simulink model "flightControlSystem"  (R2023a)
settings: Solver=ode3  StartTime=0  StopTime=TFinal  FixedStep=Ts  RelTol=1e-3  EnableMultiTasking=on
undefined symbols (not defined in the file): afterTime, codertarget, COG_X, COG_Y, Controller, corner_step, degree_range1, degree_range2, degree_range3, DiscIntNeverNeededParam, Discrete, epsilon, Estimator, g, Gamma, gray, init, modi_PI, num_threshold, over_step, prev_degree_range, prev_degree_range2, Q, R, radius, radius2, ROI_Size, rotation_degree, rotation_degree2, Sensors, straight_step, strel, Time, Ts, tuning1, tuning11, tuning2, var_acc_angle_N, var_bias_gyr_N, var_gyro_p_N, Vehicle
libraries: simulink x41, slpidlib x4, ctrlSharedLib x4, visiontransforms x4, visiontextngfix x4, sharedtransform x3, visionanalysis x3, simulink_need_slupdate x1, parrotlib x1, visionmorphops x1
(part 3 of 4)

== system flightControlSystem/Control System/State Estimator/XY Position Estimator/EstimatorXYPosition ==
  note: Switching from orientationControl to Position
      | control reset the current world position estimate
      | (happens when using no markers)
  dxy_estimin : Inport
  orient_estimin : Inport  Port=2  SampleTime=Ts
  controlModePosVSOrient_flagin : Inport  Port=3
  dz_estimin : Inport  Port=4
  Math Function : Math  Operator=transpose  SignedPower=on
  Mux2 : Mux  Inputs=2
  Product : Product  Multiplication=Matrix(*)
  Rotation Angles to Direction Cosine Matrix : sharedtransform/Rotation Angles to Direction Cosine Matrix  rotationOrder=ZYX  aMode=aMode
  SelectdXY : Selector  InputPortWidth=3  IndexOptions=Index vector (dialog)  Indices=[1 2]  OutputSizes=1
  SimplyIntegrateVelocity : DiscreteIntegrator  ExternalReset=rising  SampleTime=Ts  ICPrevOutput=DiscIntNeverNeededParam  ICPrevScaledInput=DiscIntNeverNeededParam
  XY_estimout : Outport  VectorParamsAs1DForOutWhenUnconnected=off
  wires:
  controlModePosVSOrient_flagin/1 -> SimplyIntegrateVelocity/2
  Product/1 -> SelectdXY/1
  Mux2/1 -> Product/2
  dz_estimin/1 -> Mux2/2
  SimplyIntegrateVelocity/1 -> XY_estimout/1
  dxy_estimin/1 -> Mux2/1
  orient_estimin/1 -> Rotation Angles to Direction Cosine Matrix/1
  Rotation Angles to Direction Cosine Matrix/1 -> Math Function/1
  SelectdXY/1 -> SimplyIntegrateVelocity/1
  Math Function/1 -> Product/1

== system flightControlSystem/Image Processing System/Subsystem/viewer/centroids viewer ==
  p : Inport
  In2 : Inport  Port=2
  MATLAB Function1 : MATLAB Function  TreatAsAtomicUnit=on
  MATLAB Function2 : MATLAB Function  TreatAsAtomicUnit=on
  To Workspace1 : ToWorkspace  VariableName=centroids  SampleTime=-1
  To Workspace2 : ToWorkspace  VariableName=centroids_before  SampleTime=-1
  after : VideoViewer  colormapValue=gray(256)  FigPos=[3548 573 257 231]
  before : VideoViewer  colormapValue=gray(256)  FigPos=[3816 640 285 230]
  wires:
  In2/1 -> To Workspace1/1, MATLAB Function1/1(p)
  p/1 -> MATLAB Function2/1(p), To Workspace2/1
  MATLAB Function1/1(image) -> after/1
  MATLAB Function2/1(image) -> before/1

== system flightControlSystem/Image Processing System/corner detection subsystem1/straight line detector/center line viewer ==
  center_lines : Inport
  Constant : Constant  Value=zeros(120,160)
  Draw Shapes : visiontextngfix/Draw Shapes  shape=Lines  fill=off  lineWidth=1  fillClrSource=Specify via dialog  display=White  intensity=200  color=[100 100 100 100]  opacity=0.6  viewport=Entire image  antialiasing=off  inType=Obsolete  imagePorts=One multidimensional signal  roundingMode=Floor  overflowMode=off  memoryMode=Specify word length  memoryWordLength=16  prodOutputMode=Binary point scaling  prodOutputWordLength=32  prodOutputFracLength=14  memoryFracLength=15
  center lines : VideoViewer  colormapValue=gray(256)  FigPos=[987 659 418 304]
  wires:
  Draw Shapes/1 -> center lines/1
  Constant/1 -> Draw Shapes/1
  center_lines/1 -> Draw Shapes/2

== system flightControlSystem/Image Processing System/corner detection subsystem1/straight line detector/straight line viewer ==
  Pts : Inport
  Constant : Constant  Value=zeros(120,160)
  Draw Shapes : visiontextngfix/Draw Shapes  shape=Lines  fill=off  lineWidth=1  fillClrSource=Specify via dialog  display=White  intensity=200  color=[100 100 100 100]  opacity=0.6  viewport=Entire image  antialiasing=off  inType=Obsolete  imagePorts=One multidimensional signal  roundingMode=Floor  overflowMode=off  memoryMode=Specify word length  memoryWordLength=16  prodOutputMode=Binary point scaling  prodOutputWordLength=32  prodOutputFracLength=14  memoryFracLength=15
  Straight lines : VideoViewer  colormapValue=gray(256)  FigPos=[556 648 418 304]
  wires:
  Pts/1 -> Draw Shapes/2
  Constant/1 -> Draw Shapes/1
  Draw Shapes/1 -> Straight lines/1

== system flightControlSystem/Image Processing System/corner detection1/straight line detector/center line viewer ==
  center_lines : Inport
  Constant : Constant  Value=zeros(120,160)
  Draw Shapes : visiontextngfix/Draw Shapes  shape=Lines  fill=off  lineWidth=1  fillClrSource=Specify via dialog  display=White  intensity=200  color=[100 100 100 100]  opacity=0.6  viewport=Entire image  antialiasing=off  inType=Obsolete  imagePorts=One multidimensional signal  roundingMode=Floor  overflowMode=off  memoryMode=Specify word length  memoryWordLength=16  prodOutputMode=Binary point scaling  prodOutputWordLength=32  prodOutputFracLength=14  memoryFracLength=15
  center lines : VideoViewer  colormapValue=gray(256)  FigPos=[987 659 418 304]
  wires:
  center_lines/1 -> Draw Shapes/2
  Constant/1 -> Draw Shapes/1
  Draw Shapes/1 -> center lines/1

== system flightControlSystem/Image Processing System/corner detection1/straight line detector/straight line viewer ==
  Pts : Inport
  Constant : Constant  Value=zeros(120,160)
  Draw Shapes : visiontextngfix/Draw Shapes  shape=Lines  fill=off  lineWidth=1  fillClrSource=Specify via dialog  display=White  intensity=200  color=[100 100 100 100]  opacity=0.6  viewport=Entire image  antialiasing=off  inType=Obsolete  imagePorts=One multidimensional signal  roundingMode=Floor  overflowMode=off  memoryMode=Specify word length  memoryWordLength=16  prodOutputMode=Binary point scaling  prodOutputWordLength=32  prodOutputFracLength=14  memoryFracLength=15
  Straight lines : VideoViewer  colormapValue=gray(256)  FigPos=[556 648 418 304]
  wires:
  Draw Shapes/1 -> Straight lines/1
  Constant/1 -> Draw Shapes/1
  Pts/1 -> Draw Shapes/2

== system flightControlSystem/Control System/State Estimator/SensorPreprocessing/Temperature Compensation/Triggered Subsystem ==
  In1 : Inport
  Trigger : TriggerPort  TriggerType=either  VariantControl=Variant
  Out1 : Outport
  wires:
  In1/1 -> Out1/1

== system flightControlSystem/Control System/State Estimator/XY Position Estimator/EstimatorVelocity/AccelerationHandling ==
  dxy_estimin : Inport
  sensorIMU_datin : Inport  Port=2
  orient_estimin : Inport  Port=3
  Z_estimin : Inport  Port=4
  Add : Sum  Inputs=-+
  Bus Selector1 : BusSelector  OutputSignals=ddx,ddy,ddz
  Deactivate Acceleration If OF is not used due to low altitude : simulink/Logic and Bit Operations/Compare To Constant  relop=<=  const=Estimator.pos.opticalFlowZMax  OutDataTypeStr=boolean
  Logical Operator : Logic  Operator=OR  AllPortsSameDT=off  OutDataTypeStr=boolean
  Mux6 : Mux  Inputs=3
  Product : Product  Inputs=3
  Product1 : Product  Multiplication=Matrix(*)
  Rotation Angles to Direction Cosine Matrix : sharedtransform/Rotation Angles to Direction Cosine Matrix  rotationOrder=ZYX  aMode=aMode
  SelectPlanarddxy : Selector  InputPortWidth=3  IndexOptions=Index vector (dialog)  Indices=[1 2]  OutputSizes=1
  Selector : Selector  InputPortWidth=2  IndexOptions=Index vector (dialog)  Indices=1  OutputSizes=1
  Selector1 : Selector  InputPortWidth=2  IndexOptions=Index vector (dialog)  Indices=2  OutputSizes=1
  do not use acc if optical flow never available (Note OF@60Hz but ZOH to 200!) : simulink/Logic and Bit Operations/Compare To Constant  relop=~=  const=0  OutDataTypeStr=boolean
  do not use acc if optical flow never available (Note OF@60Hz but ZOH to 200!)1 : simulink/Logic and Bit Operations/Compare To Constant  relop=~=  const=0  OutDataTypeStr=boolean
  gainaccinput1 : Gain  OutDataTypeStr=single
  gravity : Constant  Value=[0 0 -g]
  acceleration_world : Outport  OutDataTypeStr=single  VectorParamsAs1DForOutWhenUnconnected=off
  wires:
  do not use acc if optical flow never available (Note OF@60Hz but ZOH to 200!)1/1 -> Logical Operator/2
  do not use acc if optical flow never available (Note OF@60Hz but ZOH to 200!)/1 -> Logical Operator/1
  Logical Operator/1 -> Product/1
  Selector1/1 -> do not use acc if optical flow never available (Note OF@60Hz but ZOH to 200!)1/1
  Selector/1 -> do not use acc if optical flow never available (Note OF@60Hz but ZOH to 200!)/1
  dxy_estimin/1 -> Selector1/1, Selector/1
  Product/1 -> acceleration_world/1
  Deactivate Acceleration If OF is not used due to low altitude/1 -> Product/3
  Z_estimin/1 -> Deactivate Acceleration If OF is not used due to low altitude/1
  Add/1 -> SelectPlanarddxy/1
  Product1/1 -> Add/1
  gravity/1 -> Product1/2
  SelectPlanarddxy/1 -> gainaccinput1/1
  Bus Selector1/3 -> Mux6/3  "<ddz>"
  Bus Selector1/1 -> Mux6/1  "<ddx>"
  sensorIMU_datin/1 -> Bus Selector1/1
  Mux6/1 -> Add/2
  Bus Selector1/2 -> Mux6/2  "<ddy>"
  orient_estimin/1 -> Rotation Angles to Direction Cosine Matrix/1
  Rotation Angles to Direction Cosine Matrix/1 -> Product1/1
  gainaccinput1/1 -> Product/2

== system flightControlSystem/Control System/State Estimator/XY Position Estimator/EstimatorVelocity/Angular velocity compensation for optical flow ==
  note: Optical flow readings are affected by both linear and angular velocity of the drone. We need to subtract the effect of angular velocity before using the flow data
  z_estimate : Inport
  Angular velocity w/o bias : Inport  Port=2
  Abs : Abs  SaturateOnIntegerOverflow=off
  Data Type Conversion : DataTypeConversion  SaturateOnIntegerOverflow=off  RndMeth=Floor
  Demux : Demux  Outputs=2
  Gain1 : Gain  Gain=-1
  Mux : Mux  Inputs=2
  Selector : Selector  InputPortWidth=3  IndexOptions=Index vector (dialog)  Indices=[1 2]  OutputSizes=1
  prod : Product  Inputs=**
  angular velocity correction : Outport
  wires:
  Gain1/1 -> Mux/1
  Mux/1 -> Data Type Conversion/1
  Demux/2 -> Gain1/1
  Data Type Conversion/1 -> angular velocity correction/1
  prod/1 -> Demux/1
  z_estimate/1 -> Abs/1
  Demux/1 -> Mux/2
  Selector/1 -> prod/2
  Abs/1 -> prod/1
  Angular velocity w/o bias/1 -> Selector/1

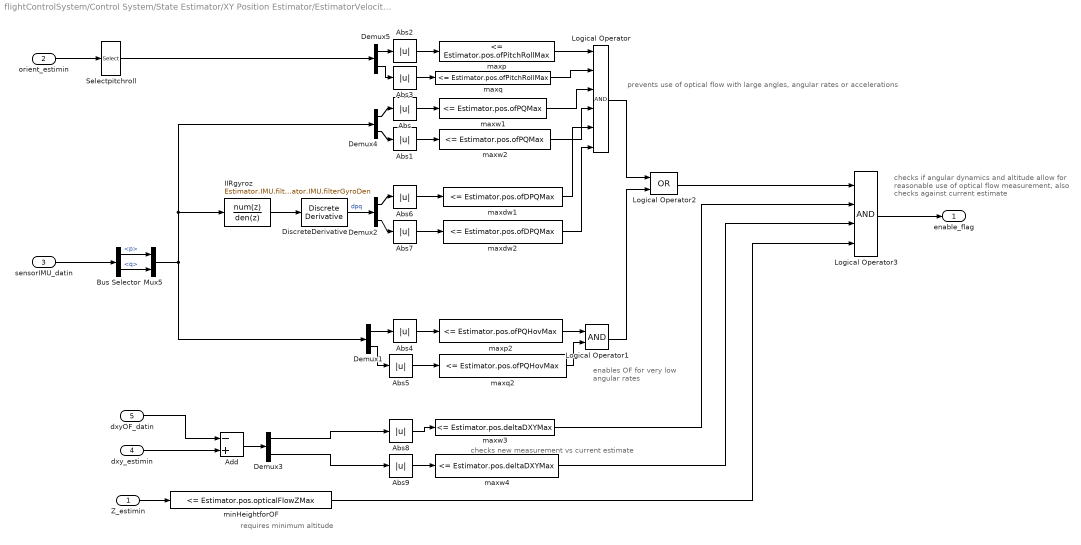
== system flightControlSystem/Control System/State Estimator/XY Position Estimator/EstimatorVelocity/DataHandling ==
  note: prevents use of optical flow with large angles, angular rates or accelerations
  note: enables OF for very
      | low angular rates
  note: checks if angular dynamics and altitude allow for
      | reasonable use of optical flow measurement,
      | also checks against current estimate
  note: checks new measurement vs current estimate
  note: requires minimum altitude
  Z_estimin : Inport
  orient_estimin : Inport  Port=2
  sensorIMU_datin : Inport  Port=3
  dxy_estimin : Inport  Port=4
  dxyOF_datin : Inport  Port=5
  Abs{,1..9} (10 alike) : Abs  SaturateOnIntegerOverflow=off
  Add : Sum  Inputs=-+
  Bus Selector : BusSelector  OutputSignals=p,q
  Demux{1..5} (5 alike) : Demux  Outputs=2
  DiscreteDerivative : simulink/Discrete/Discrete Derivative  gainval=1.0  ICPrevScaledInput=0.0  OutMin=[]  OutMax=[]  OutDataType=fixdt(1, 16)  OutScaling=2^-10  DoSatur=off
  IIRgyroz : DiscreteFilter  Numerator=Estimator.IMU.filterGyroNum  Denominator=Estimator.IMU.filterGyroDen
  Logical Operator : Logic  Inputs=6  AllPortsSameDT=off  OutDataTypeStr=boolean
  Logical Operator1 : Logic  AllPortsSameDT=off  OutDataTypeStr=boolean
  Logical Operator2 : Logic  Operator=OR  AllPortsSameDT=off  OutDataTypeStr=boolean
  Logical Operator3 : Logic  Inputs=4  AllPortsSameDT=off  OutDataTypeStr=boolean
  Mux5 : Mux  Inputs=2
  Selectpitchroll : Selector  InputPortWidth=3  IndexOptions=Index vector (dialog)  Indices=[2 3]  OutputSizes=1
  maxdw1 : simulink/Logic and Bit Operations/Compare To Constant  relop=<=  const=Estimator.pos.ofDPQMax  OutDataTypeStr=boolean
  maxdw2 : simulink/Logic and Bit Operations/Compare To Constant  relop=<=  const=Estimator.pos.ofDPQMax  OutDataTypeStr=boolean
  maxp : simulink/Logic and Bit Operations/Compare To Constant  relop=<=  const=Estimator.pos.ofPitchRollMax  OutDataTypeStr=boolean
  maxp2 : simulink/Logic and Bit Operations/Compare To Constant  relop=<=  const=Estimator.pos.ofPQHovMax  OutDataTypeStr=boolean
  maxq : simulink/Logic and Bit Operations/Compare To Constant  relop=<=  const=Estimator.pos.ofPitchRollMax  OutDataTypeStr=boolean
  maxq2 : simulink/Logic and Bit Operations/Compare To Constant  relop=<=  const=Estimator.pos.ofPQHovMax  OutDataTypeStr=boolean
  maxw1 : simulink/Logic and Bit Operations/Compare To Constant  relop=<=  const=Estimator.pos.ofPQMax  OutDataTypeStr=boolean
  maxw2 : simulink/Logic and Bit Operations/Compare To Constant  relop=<=  const=Estimator.pos.ofPQMax  OutDataTypeStr=boolean
  maxw3 : simulink/Logic and Bit Operations/Compare To Constant  relop=<=  const=Estimator.pos.deltaDXYMax  OutDataTypeStr=boolean
  maxw4 : simulink/Logic and Bit Operations/Compare To Constant  relop=<=  const=Estimator.pos.deltaDXYMax  OutDataTypeStr=boolean
  minHeightforOF : simulink/Logic and Bit Operations/Compare To Constant  relop=<=  const=Estimator.pos.opticalFlowZMax  OutDataTypeStr=boolean
  enable_flag : Outport  VectorParamsAs1DForOutWhenUnconnected=off
  wires:
  minHeightforOF/1 -> Logical Operator3/4
  IIRgyroz/1 -> DiscreteDerivative/1
  Mux5/1 -> Demux1/1, Demux4/1, IIRgyroz/1
  maxw4/1 -> Logical Operator3/3
  maxw3/1 -> Logical Operator3/2
  dxyOF_datin/1 -> Add/1
  Demux3/2 -> Abs9/1
  Demux3/1 -> Abs8/1
  dxy_estimin/1 -> Add/2
  Add/1 -> Demux3/1
  Abs9/1 -> maxw4/1
  Abs8/1 -> maxw3/1
  Logical Operator2/1 -> Logical Operator3/1
  Logical Operator3/1 -> enable_flag/1
  DiscreteDerivative/1 -> Demux2/1  "dpq"
  Demux2/2 -> Abs7/1
  Demux2/1 -> Abs6/1
  Abs7/1 -> maxdw2/1
  Abs6/1 -> maxdw1/1
  Logical Operator1/1 -> Logical Operator2/2
  Demux1/2 -> Abs5/1
  Demux1/1 -> Abs4/1
  Abs5/1 -> maxq2/1
  Abs4/1 -> maxp2/1
  Abs3/1 -> maxq/1
  Abs2/1 -> maxp/1
  Demux4/2 -> Abs1/1
  Demux4/1 -> Abs/1
  Abs1/1 -> maxw2/1
  Abs/1 -> maxw1/1
  Z_estimin/1 -> minHeightforOF/1
  Logical Operator/1 -> Logical Operator2/1
  maxw1/1 -> Logical Operator/3
  Bus Selector/1 -> Mux5/1  "<p>"
  Selectpitchroll/1 -> Demux5/1
  sensorIMU_datin/1 -> Bus Selector/1
  maxq2/1 -> Logical Operator1/2
  Bus Selector/2 -> Mux5/2  "<q>"
  maxp/1 -> Logical Operator/1
  maxw2/1 -> Logical Operator/4
  orient_estimin/1 -> Selectpitchroll/1
  maxdw1/1 -> Logical Operator/5
  maxdw2/1 -> Logical Operator/6
  maxq/1 -> Logical Operator/2
  Demux5/1 -> Abs2/1
  Demux5/2 -> Abs3/1
  maxp2/1 -> Logical Operator1/1

== system flightControlSystem/Control System/State Estimator/XY Position Estimator/EstimatorVelocity/xy velocity w//o angular velocity compensation ==
  note: Optical flow raw readings are converted to velocity in m/s based on the estimated altitude
  optical_flow : Inport
  z_estimate : Inport  Port=2
  " " : Product  Inputs=**
  Compare To Constant : simulink/Logic and Bit Operations/Compare To Constant  relop=<  const=200*4  OutDataTypeStr=boolean
  Counter Free-Running : simulink/Sources/Counter Free-Running  NumBits=32  tsamp=-1
  Gain : Gain  Gain=-1
  Select dxy : Selector  InputPortWidth=3  IndexOptions=Index vector (dialog)  Indices=[1 2]  OutputSizes=1
  Switch : Switch  Criteria=u2 > Threshold  SaturateOnIntegerOverflow=off  InputSameDT=off
  opticalFlowErrorCorrect : Gain  Gain=1.15
  optical_flow_dx_dy : Outport
  wires:
  Select dxy/1 -> optical_flow_dx_dy/1  "optical_flow_dx_dy"
  " "/1 -> opticalFlowErrorCorrect/1
  opticalFlowErrorCorrect/1 -> Switch/3
  Gain/1 -> " "/2
  Switch/1 -> Select dxy/1
  Counter Free-Running/1 -> Compare To Constant/1
  Compare To Constant/1 -> Switch/2
  optical_flow/1 -> " "/1, Switch/1
  z_estimate/1 -> Gain/1

== matlab function flightControlSystem/Image Processing System/Subsystem/calculate yaw ==
  data: u input; yaw output
function yaw = fcn(u)

p = u(2,:);

yaw = mod(atan2(p(2),p(1)) , 2*pi);

if yaw > pi
   yaw =  yaw- 2*pi; 
end

== matlab function flightControlSystem/Control System/Controller/Position Controller/Position error transformation (Earth to Body frame) ==
  data: yaw input; xy_err_earth input; xy_err_body output
function xy_err_body = fcn(yaw,xy_err_earth)

transformation = [cos(yaw), sin(yaw); -sin(yaw),  cos(yaw)];
xy_err_body = transformation * xy_err_earth;


end

== matlab function flightControlSystem/Image Processing System/Subsystem/viewer/centroids viewer/MATLAB Function1 ==
  data: p input; image output
function image = fcn(p)

image = zeros(120, 160);

for i = 1:5
    if( p(i,1) == 0)  || (p(i,2) == 0)
       continue; 
    end
    x = round(p(i,1));
    y = round(p(i,2));
    image(x,y) = 1;
end

== matlab function flightControlSystem/Image Processing System/Subsystem/viewer/centroids viewer/MATLAB Function2 ==
  data: p input; image output
function image = fcn(p)

image = zeros(120, 160);


for i = 1:5
    if( p(i,1) == 0)  || (p(i,2) == 0)
       continue; 
    end
    x = round(p(i,1));
    y = round(p(i,2));
    image(x,y) = 1;
end

== matlab function flightControlSystem/Control System/Path Planning/mpc/Triggered Subsystem/discrete_MPC ==
  data: input input; vx output; vy output; corner input; modi_PI input; R input; Q input; epsilon input; Gamma input; landing input; corner_step input; straight_step input
function [vx,vy]  = discrete_mpc(input,corner,modi_PI,R,Q,epsilon,Gamma, landing, corner_step, straight_step)
if landing==1
    vx=input(10);
    vy=input(11);
    return;
end


if corner==1
    step=corner_step;
else
    step=straight_step;
end
tic
%DISCRETE_MPC
% coder.extrinsic('quadprog');
%using drone dynamics
%result=[phi theta pi p q r u v w x y z];
Horizon =10;
x=input(1:12);
x_d=input(12+Horizon);
y_d=input(12+2*Horizon);
z_d=1.3;
dt=1;
desti=[0 0 0 0 0 0 0 0 0 x_d y_d z_d]';%destination
real_x=x(10);
real_y=x(11);
real_z=x(12);
dx=(x_d-real_x)/Horizon;
dy=(y_d-real_y)/Horizon;
dz=(z_d-real_z)/Horizon;
% reference making
desti_horizon=zeros(12*Horizon,1);
ref_const=zeros(12*Horizon,1);
for i=1:Horizon
    %    desti_horizon=[desti_horizon;[0 0 0 0 0 0 0 0 0 real_x+dx*i real_y+dy*i real_z+dz*i]'];
    desti_horizon(10+(i-1)*12)=x_d;
    desti_horizon(11+(i-1)*12)=y_d;
    desti_horizon(12+(i-1)*12)=z_d;
%     desti_horizon=[desti_horizon;[0 0 0 0 0 0 0 0 0 real_x+dx*(i) real_y+dy*(i) real_z+dz*(i)]'];
    ref_const(10+(i-1)*12)=input(12+i);
    ref_const(11+(i-1)*12)=input(12+Horizon+i);
end

%% quadprog

H=R+modi_PI'*Q*modi_PI;
f=((x)'*Gamma'*Q*modi_PI-desti_horizon'*Q*modi_PI);
xmax=repmat(1000000000,12*Horizon,1);
xmin=repmat(-100000000,12*Horizon,1);
u_max=repmat([10,10,10,10,10,10,10,10,10,1000,1000,1000,1,5,5,5]',Horizon,1);
u_min=repmat(-[10,10,10,50,50,50,50,50,50,1000,1000,1000,1,.001,.001,0.0011]',Horizon,1);
%U=quadprog(H,f',[eye(320);-eye(320);PI;-PI],[u_max;-u_min;(xmax)-Gamma*(x); (-xmin)+Gamma*(x)]);
temp_PI=zeros(Horizon*12,Horizon*16);
temp_ref=zeros(12*Horizon,1);
epsilon_r=zeros(12*Horizon,1);
for i=1:Horizon
    temp_PI(12*(i-1)+10,:)=modi_PI(12*(i-1)+10,:);
    temp_PI(12*(i-1)+11,:)=modi_PI(12*(i-1)+11,:);
    temp_PI(12*(i-1)+12,:)=modi_PI(12*(i-1)+12,:);
    temp_ref(12*(i-1)+10)=ref_const(12*(i-1)+10);
    temp_ref(12*(i-1)+11)=ref_const(12*(i-1)+11);
    temp_ref(12*(i-1)+12)=ref_const(12*(i-1)+12);
    epsilon_r(12*(i-1)+10)=epsilon(10);
    epsilon_r(12*(i-1)+11)=epsilon(11);
    epsilon_r(12*(i-1)+12)=epsilon(12);
end
temp_x=[0 0 0 0 0 0 0 0 0 x(10) x(11) 0]';
opts = optimoptions('quadprog','Algorithm','active-set');
% opts = optimoptions(opts,'MaxIterations',1e4); % Recommended
x0=zeros(16*Horizon,1);
% for i=1:Horizon
%    x0(1+16*(i-1))=x_esti(1);
%    x0(2+16*(i-1))=x_esti(2);
%    x0(3+16*(i-1))=x_esti(3);
%    x0(4+16*(i-1))=x_esti(4);
%    x0(5+16*(i-1))=x_esti(5);
%    x0(6+16*(i-1))=x_esti(6);
%    x0(7+16*(i-1))=x_esti(7);
%    x0(8+16*(i-1))=x_esti(8);
%    x0(9+16*(i-1))=x_esti(9);
%    x0(10+16*(i-1))=x_esti(10);
%    x0(11+16*(i-1))=x_esti(11);
%    x0(12+16*(i-1))=x_esti(12);
%    x0(13+16*(i-1))=0;
%    x0(14+16*(i-1))=0;
%    x0(15+16*(i-1))=0;
%    x0(16+16*(i-1))=0;
% end
for i=1:Horizon
   x0(1+16*(i-1))=x(1);
   x0(2+16*(i-1))=x(2);
   x0(3+16*(i-1))=x(3);
   x0(4+16*(i-1))=x(4);
   x0(5+16*(i-1))=x(5);
   x0(6+16*(i-1))=x(6);
   x0(7+16*(i-1))=x(7);
   x0(8+16*(i-1))=x(8);
   x0(9+16*(i-1))=x(9);
   x0(10+16*(i-1))=x(10);
   x0(11+16*(i-1))=x(11);
   x0(12+16*(i-1))=x(12);
   x0(13+16*(i-1))=0;
   x0(14+16*(i-1))=0;
   x0(15+16*(i-1))=0;
   x0(16+16*(i-1))=0;
end
U=zeros(16*Horizon,1);
U=quadprog(H,f',[eye(16*Horizon);-eye(16*Horizon);temp_PI;-temp_PI],[u_max;-u_min;(temp_ref+epsilon_r)-Gamma*(temp_x); (-(temp_ref-epsilon_r))+Gamma*(temp_x)],[],[],[],[],x0,opts);
y=zeros(12*Horizon,1);
y=Gamma*x+modi_PI*U;
a=12*step+10;
b=12*step+11;
vx = y(a);
vy = y(b);
toc
end

== stateflow chart flightControlSystem/Image Processing System/Chart ==
  state take_off
    entry:
    takeOffFlag= 0;
    refPosition1 = [0 0];
  state take_off_complete
    entry, during:
    [refPosition1, theta] = init(preprocessingDots);
    isStraightLine = 1;
  state straight_line_reference_generation
    entry:
    isLine = 1;
    during:
    tempPoint = zeros(1,2);
    [isLine, tempPoint, cutting_image] = sector_form(preprocessingDots, theta);
    [refPosition1, theta] = reference_generator(tempPoint);
    tempPoint2 =second_track_generator(preprocessingDots,  refPosition1);
    [refPosition2, theta2] = reference_generator(tempPoint2);
  state new_track_generation
    entry:
    isLine = 0;
    isLanding = 0;
    tempRef = zeros(1,2);
    during:
    state state_check
      [isLanding, tempRef,cntt,MAPP] = laning_check(ladingFlag, theta,landingDots);
    state asd
      tempPoint =track_generator(preprocessingDots,theta);
      [refPosition1, theta] = reference_generator(tempPoint);
      tempPoint2 =second_track_generator(preprocessingDots,  refPosition1);
      [refPosition2, theta2] = reference_generator(tempPoint2);
      isLine = 1;
    (default) -> state_check
    state_check -> asd
  state landing
    entry,during:
    during:
    %[isLanding, refPosition1,cntt,MAPP] = laning_check(ladingFlag, theta,landingDots);
    %refPosition2 = refPosition1;
    refPosition1=landingRef;
    refPosition2=landingRef;
  (default) -> take_off
  take_off -> take_off_complete : [abs(Z)  >  1.3]
  take_off_complete -> straight_line_reference_generation : [1]
  straight_line_reference_generation -> new_track_generation : after(afterTime,sec)[isLine == 0]
  new_track_generation -> straight_line_reference_generation [order 1] : [isLanding ==0 && isLine == 1]
  new_track_generation -> landing [order 2] : [isLanding == 1]
  data: points function_input; initial_ref function_output; initial_theta function_output; state function_output; ref function_output; points function_input; prev_theta function_input; MAP function_output; num_threshold parameter; degree_range1 parameter; points function_input; ref function_output; degree_range2 parameter; rotation_degree parameter; prev_degree_range parameter; radius parameter; prev_theta function_input; image function_input; dot function_input; point function_output; ref function_output; newTheta function_output; point function_input; points function_input; ref function_output; degree_range3 parameter; rotation_degree2 parameter; radius2 parameter; prev_degree_range2 parameter; rotationCenter function_input; flag function_input; curTheta function_input; state function_output; ref function_output; points function_input; COG_Y parameter; COG_X parameter; cnt function_output; MAP function_output; ROI_Size parameter; takeOffFlag local; refPosition1 output; refPosition2 output; preprocessingDots input; isLine local; COG_X constant double =60; COG_Y constant double =80; tempPoint local; ladingFlag input; theta local; tempPoint2 local; theta2 local; isLanding output; cutting_image output; Z input; tempRef local; isStraightLine local; afterTime parameter; landingDots input; cntt output; MAPP output; landingRef input
  function [initial_ref, initial_theta] = init(points):
    | function [initial_ref, initial_theta] = init(points)
    | 
    | % mean calculate
    | points(points==0) = NaN;
    | initial_ref = mean(points,1,'omitnan');
    | 
    | % cordinate change
    | initial_ref(1) = COG_X - initial_ref(1);
    | initial_ref(2) = initial_ref(2) - COG_Y;
    | 
    | % initial theta calculate
    | initial_theta = mod(atan2(initial_ref(2) ,initial_ref(1) ),2*pi);
  function [state,ref, MAP]= sector_form(points, prev_theta):
    | function [state,ref, MAP]= sector_form(points, prev_theta)
    | 
    | num_dots = size(points,1);
    | cutting_dots = zeros(num_dots,2);
    | ref = zeros(1,2);
    | cnt = 0;
    | MAP=zeros(120,160);
    | 
    | for i=1:num_dots
    |     %탈출조건
    |     if points(i,1) == 0
    |        break; 
    |     end
    |     % 0~180도 사이의 각만 추출
    |     delta = abs( mod(atan2(points(i,2)-COG_Y, COG_X-points(i,1)),2*pi)  -  prev_theta);
    |     if delta > pi
    |         delta = 2*pi - delta;
    |     end
    |     
    |     if  delta< deg2rad(degree_range1 * 0.5)
    |         cnt = cnt+1;
    |         cutting_dots(cnt,1) = points(i,1);
    |         cutting_dots(cnt,2) = points(i,2);
    |         MAP(points(i,1),points(i,2))=1;
    |     end
    | end
    | 
    | 
    | % %라벨 붙여서 해결하기
    | % pre_dist = Inf;
    | % center = ones(1,2);
    | % for i = 1:cnt
    | %     dist = norm( cutting_dots(i,:) - [COG_X, COG_Y]);
    | %     if dist < pre_dist
    | %         center = cutting_dots(i,:);
    | %         pre_dist = dist;
    | %     end
    | % end
    | % L_image = bwlabel(MAP,8);
    | % label = L_image(center(1,1), center(1,2) );
    | % seg_image = L_image==label;
    | % 
    | % cnt = 0;
    | % cutting_dots = zeros(num_dots,2);
    | % for i = 1:120
    | %    for j = 1:160
    | %       if  seg_image(i,j) == 1
    | %           cnt = cnt+1;
    | %           cutting_dots(cnt,1) = i;
    | %           cutting_dots(cnt,2) = j;
    | %       end
    | %    end
    | % end
    | cutting_dots(cutting_dots==0) = NaN;
    | ref = mean(cutting_dots,1,'omitnan');
    | 
    | % Line인지 아닌지 판단
    | if cnt > num_threshold
    |     state = 1;
    | else
    |     state = 0;
    | end
    | 
    | % if cnt > straight_threshold
    | %     straight_state = 1;
    | % else
    | %     straight_state = 0;
    | % end
    | 
    | 
    | 
    | % cutting_dots(cutting_dots==0) = NaN;
    | % rho = 4*2; % tunning
    | % diagonal = 100;
    | % iterator = ceil(diagonal/rho);
    | % R = 5; %tunning
    | % theta = pi - prev_theta; % frame좌표로 변환
    | % P = zeros(1,2);
    | % cornerFalg = 0;
    | % radius = 0;
    | % for k = 0:iterator
    | %      P = [COG_X, COG_Y] + k * [rho*cos(prev_theta), rho*sin(prev_theta)];
    | %      if isempty( rangesearch(cutting_dots,P,R) )
    | %          radius = rho*k;
    | %      end
    | % end
    | % 
    | % num = 0;
    | % for i=1:cnt
    | %     % NaN때문에 여기서 에러 날수도?
    | %     if isnan(cutting_dots(i,:))
    | %        break; 
    | %     end
    | %    if norm(cutting_dots(i,:) - [COG_X, COG_Y]) > radius
    | %        cutting_dots(i,:) = NaN;
    | %        num = num + 1;
    | %    end
    | % end
    | % ref = mean(cutting_dots,1,'omitnan');
    | % 
    | % cnt = cnt - num;
    | % if cnt > num_threshold
    | %     state = 1;
    | % else
    | %     state = 0;
    | % end
    | % %여기서 state = 0이 계속 타지네... 흠흠..!@#!@#@!#!
    | 
    | 
    | 
    | 
    | % % % se = strel('disk',3);
    | % % % MAP = imdilate(MAP, se);
    | % % % pre_dist = Inf;
    | % % % center = ones(1,2);
    | % % % for i = 1:cnt
    | % % %     dist = norm( cutting_dots(i,:) - [COG_X, COG_Y]);
    | % % %     if dist < pre_dist
    | % % %         center = cutting_dots(i,:);
    | % % %         pre_dist = dist;
    | % % %     end
    | % % % end
    | % % % L_image = bwlabel(MAP,8);
    | % % % label = L_image(center(1,1), center(1,2) );
    | % % % seg_image = L_image==label;
    | % % % 
    | % % % cnt = 0;
    | % % % cutting_dots = zeros(num_dots,2);
    | % % % for i = 1:120
    | % % %    for j = 1:160
    | % % %       if  seg_image(i,j) == 1
    | % % %           cnt = cnt+1;
    | % % %           cutting_dots(cnt,1) = i;
    | % % %           cutting_dots(cnt,2) = j;
    | % % %       end
    | % % %    end
    | % % % end
    | % % % cutting_dots(cutting_dots==0) = NaN;
    | % % % ref = mean(cutting_dots,1,'omitnan');
    | % % 
    | % % 
    | % % % I = find(seg_image==1);
    | % % % [row, col] = ind2sub(size(seg_image), I);
    | % % % dotss = zeros(2000,2);
    | % % % for i= 1:size(row)
    | % % %     dotss = [row(i), col(i)];
    | % % % end
    | % % % dotss(dotss==0) = NaN;
    | % % % ref = mean(dotss,1,'omitnan');
    | % % 
    | % % 
    | % % % 일정한 호 이내의 점 추출 (방법이 잘못 된듯)
    | % % % r1 = 20;
    | % % % r2 = 30;
    | % % % arcPoints = zeros(100,2);
    | % % % idx = 1;
    | % % % for i = 1:num_dots
    | % % %     if cutting_dots(i,1) == 0
    | % % %        break; 
    | % % %     end
    | % % %     R = sqrt( (cutting_dots(i,1) - COG_X)^2 + (cutting_dots(i,2) - COG_Y)^2 ) ;
    | % % %     if R>=r1 && R<=r2
    | % % %         arc_cnt = arc_cnt + 1;
    | % % %     end
    | % % %     if R <= r1
    | % % %         arcPoints(idx,1) = cutting_dots(i,1);
    | % % %         arcPoints(idx,2) = cutting_dots(i,2);
    | % % %         idx = idx+1;
    | % % %     end  
    | % % % end
    | % % % 
    | % % % if arc_cnt > arc_threshold
    | % % %     cutting_dots(cutting_dots==0) = NaN;
    | % % %     ref = mean(cutting_dots,1,'omitnan');
    | % % % else
    | % % %     arcPoints(arcPoints==0) = NaN;
    | % % %     ref = mean(arcPoints,1,'omitnan');
    | % % % end
    | % % 
    | % % 
    | % % % % clustering
    | % % % temp_dist = 0;
    | % % % p = zeros(1,2);
    | % % % center = [60, 80];
    | % % % for i = 1:num_dots
    | % % %     if cutting_dots(i,1) == 0
    | % % %         break;
    | % % %     end
    | % % %    dist = norm( center - cutting_dots(1,:) );  
    | % % %    if dist > temp_dist
    | % % %        p = cutting_dots(i,:);
    | % % %        temp_dist = dist;
    | % % %    end
    | % % % end
    | % % % centroids = [center ; p];
    | % % % idx = knnsearch(centroids,cutting_dots);
    | % % % cutting_dots(cutting_dots==0) = NaN;
    | % % % ref = mean(cutting_dots(idx==1,:),1,'omitnan');
  function ref  = track_generator(points, prev_theta):
    | function ref  = track_generator(points, prev_theta)
    | num_dots = size(points,1);
    | cutting_dots = zeros(num_dots,2);
    | iterator = round(360 / rotation_degree);
    | prev_theta = mod(prev_theta+ pi , 2*pi);
    | 
    | cnt = 1;
    | ref = zeros(1,2);
    | plus_degree = (prev_degree_range/2) + (degree_range2/2);
    | iterator = round( (360 - 2*plus_degree) / rotation_degree );
    | pre_cnt = 0;
    | for i = 0:iterator
    |     cutting_dots = zeros(num_dots,2);
    |     cnt = 0;
    |     for j=1:num_dots
    |         %탈출조건
    |         if points(j,1) == 0
    |            break;
    |         end
    |         % 0~180도 사이의 각만 추출
    |         %delta = abs( mod(atan2(points(j,2)-COG_Y, COG_X-points(j,1)),2*pi)  -  mod(prev_theta + i*deg2rad(rotation_degree) , 2*pi) );
    |         delta = abs( mod(atan2(points(j,2)-COG_Y, COG_X-points(j,1)),2*pi)  -  mod(prev_theta + deg2rad(plus_degree) +i*deg2rad(rotation_degree) , 2*pi) );
    |         if delta > pi
    |             delta = 2*pi - delta;
    |         end
    |         R = sqrt( (points(j,1) - COG_X)^2 + (points(j,2) - COG_Y)^2 ) ;
    |         % degree_range 이내 && radius이내 점 추출
    |         if  delta< deg2rad(degree_range2 * 0.5) && R < radius
    |             cnt = cnt+1;
    |             cutting_dots(cnt,1) = points(j,1);
    |             cutting_dots(cnt,2) = points(j,2);
    |         end
    |     end
    |     if cnt > pre_cnt
    |         cutting_dots(cutting_dots==0) = NaN;
    |         ref = mean(cutting_dots,1,'omitnan');
    |         pre_cnt = cnt;
    |     end
    | end
  function point = means_circle(image, dot):
    | function point = means_circle(image, dot)
    | 
    | r = 30;
    | 
    | % dot을 pixel좌표로 변환
    | % dot(1) = COG_X - dot(1);
    | % dot(2) = dot(2) + COG_Y;
    | 
    | % boundary processing
    | if dot(1) -r < 1
    |    startX = 1;
    | else
    |     startX = dot(1) -r;
    | end
    |     
    | if dot(2) -r < 1
    |    startY = 1;
    | else
    |     startY = dot(2) -r;
    | end
    | 
    | if dot(1) + r > 120
    |     endX = 120;
    | else
    |     endX = dot(1) + r;
    | end
    | 
    | if dot(2) + r > 160
    |     endY = 160;
    | else
    |     endY = dot(2) + r;
    | end
    |     
    | startPonit = [startX, startY];
    | endPoint = [endX, endY];
    | 
    | % k-means
    | ROIdots = zeros(2000,2);
    | idx = 1;
    | 
    | for i = round(startX) : round(endX)
    |     for j = round(startY) : round(endY)
    |        if image(i,j) == 1
    |            dist = sqrt( (dot(1) - i)^2 + (dot(2) - j)^2  );
    |            if dist <= r
    |               ROIdots(idx,1) = i;
    |               ROIdots(idx,2) = j;
    |               idx = idx+1;
    |            end
    |        end
    |     end
    | end
    | 
    | ROIdots(ROIdots==0) = NaN;
    | point = mean(ROIdots,1,'omitnan');
  function [ref, newTheta] = reference_generator(point):
    | function [ref, newTheta] = reference_generator(point)
    | 
    | ref = zeros(1,2);
    | ref(1) = COG_X - point(1);
    | ref(2) = point(2) - COG_Y;
    | newTheta = mod(atan2(ref(2) ,ref(1) ),2*pi);
  function ref  = second_track_generator(points, rotationCenter):
    | function ref  = second_track_generator(points, rotationCenter)
    | 
    | num_dots = size(points,1);
    | cutting_dots = zeros(num_dots,2);
    | iterator = round(360 / rotation_degree2);
    | prev_theta = mod(atan2( 0 - rotationCenter(2) , 0 - rotationCenter(1) ),2*pi);
    | cnt = 1;
    | ref = zeros(1,2);
    | 
    | plus_degree = (prev_degree_range2/2) + (degree_range3/2); 
    | iterator = round( (360 - 2*plus_degree) / rotation_degree2 );
    | 
    | 
    | pre_cnt = 0;
    | for i = 0:iterator
    |     cutting_dots = zeros(num_dots,2);
    |     cnt = 1;
    |     for j=1:num_dots
    |         %탈출조건
    |         if points(j,1) == 0
    |            break; 
    |         end
    |         % 0~180도 사이의 각만 추출
    |         P = [COG_X-points(j,1), points(j,2)-COG_Y];
    |         delta = abs( mod(atan2(P(2) - rotationCenter(2) , P(1) - rotationCenter(1) ),2*pi)  -  mod(prev_theta + deg2rad(plus_degree) +i*deg2rad(rotation_degree2) , 2*pi) );
    |         if delta > pi
    |             delta = 2*pi - delta;
    |         end
    |         R = sqrt( (P(1) - rotationCenter(1))^2 + (P(2) - rotationCenter(2))^2 ) ;
    |         % degree_range 이내 && radius이내 점 추출
    |         if  delta< deg2rad(degree_range3 * 0.5) && R < radius2
    |             cutting_dots(cnt,1) = points(j,1);
    |             cutting_dots(cnt,2) = points(j,2);
    |             cnt = cnt+1;
    |         end
    |     end
    |     
    |     if cnt > pre_cnt 
    |         cutting_dots(cutting_dots==0) = NaN;
    |         ref = mean(cutting_dots,1,'omitnan');
    |         pre_cnt = cnt;
    |     end
    |     
    | end
  function [state, ref,cnt, MAP] = laning_check(flag, curTheta, points):
    | function [state, ref,cnt, MAP] = laning_check(flag, curTheta, points)
    | 
    | num_dots = size(points,1);
    | cutting_dots = zeros(num_dots,2);
    | ref = zeros(1,2);
    | cnt = 0;
    | landing_threshold = 10;
    | MAP=zeros(120,160);
    | 
    | for i=1:num_dots
    |     %탈출조건
    |     if points(i,1) == 0
    |        break; 
    |     end
    |     % 0~180도 사이의 각만 추출
    |     delta = abs( mod(atan2(points(i,2)-(ROI_Size/2), (ROI_Size/2)-points(i,1)),2*pi)  -  curTheta);
    |     if delta > pi
    |         delta = 2*pi - delta;
    |     end
    |     
    |     if  delta< deg2rad(90 * 0.5)
    |         cnt = cnt+1;
    |         cutting_dots(cnt,1) = points(i,1);
    |         cutting_dots(cnt,2) = points(i,2);
    |         MAP(points(i,1),points(i,2))=1;
    |     end
    | end
    | 
    | 
    | state = 0;
    | 
    | if flag == 1 && cnt > landing_threshold
    |     cutting_dots(cutting_dots==0) = NaN;
    |     ref = mean(cutting_dots,1,'omitnan');
    |     ref(1) = (ROI_Size/2) - ref(1);
    |     ref(2) = ref(2) - (ROI_Size/2);
    |     
    |     state = 1;
    | else
    |     state = 0;
    | end
    | 
    | % landingTheta = mod(atan2(landing_ref(2), landing_ref(1)), 2*pi);
    | % deltaTheta = abs(mod(landingTheta - curTheta, 2*pi));
    | % if deltaTheta > pi
    | %             deltaTheta = 2*pi - deltaTheta;
    | % end
    | % 
    | % if flag == 1 && deltaTheta < deg2rad(30 * 0.5)
    | %     state = 1;
    | %     ref = landing_ref;
    | % end

== matlab function flightControlSystem/Image Processing System/preprocessing subsystem/Line segment ==
  data: dots input; MAP input; seg_image output; COG_X parameter; COG_Y parameter
function seg_image  = fcn(dots, MAP,COG_X, COG_Y)


num_dots = size(dots,1);

tmep_dist = Inf;
center = ones(1,2);
for i = 1:num_dots
    if dots(i,1) == 0
        break;
    end
    dist = norm( dots(i,:) - [COG_X, COG_Y]);
    if dist < tmep_dist
        center = dots(i,:);
        tmep_dist = dist;
    end
end


L_image = bwlabel(MAP,8);
label = L_image(center(1,1), center(1,2) );
seg_image = L_image==label;

cnt = 0;
cutting_dots = zeros(num_dots,2);
for i = 1:120
   for j = 1:160
      if  seg_image(i,j) == 1
          cnt = cnt+1;
          cutting_dots(cnt,1) = i;
          cutting_dots(cnt,2) = j;
      end
   end
end

== matlab function flightControlSystem/Image Processing System/Subsystem1/MATLAB Function2 ==
  data: X input; prev_points output; Y input; COG_X parameter; COG_Y parameter; MAP output
function [prev_points,MAP] = fcn(X, Y,COG_X, COG_Y)
persistent X1 X2 X3 Y1 Y2 Y3
if isempty(X1)
    X1 = 0;
end
if isempty(X2)
    X2 = 0;
end
if isempty(X3)
    X3 = 0;
end
if isempty(Y1)
    Y1 = 0;
end
if isempty(Y2)
    Y2 = 0;
end
if isempty(Y3)
    Y3 = 0;
end
prev_points = [COG_X-(X1-X)*2000 COG_Y+(Y1-Y)*2000;COG_X-(X2-X)*2000 COG_Y+(Y2-Y)*2000;COG_X-(X3-X)*2000 COG_Y+(Y3-Y)*2000];
prev_points = round(prev_points);
X3 = X2; Y3 = Y2;
X2 = X1; Y2 = Y1;
X1 = X; Y1 = Y;
MAP = zeros(120,160);
for i=1:3
    if 1<=prev_points(i,1) && prev_points(i,1)<=120 && 1<=prev_points(i,2) && prev_points(i,2)<=160 
        MAP(prev_points(i,1),prev_points(i,2))=1;
    end
end

== matlab function flightControlSystem/Image Processing System/preprocessing subsystem/preprocessing ==
  data: bin_image input; ref_image output; preporcessingDots output
function [ref_image, preporcessingDots]  = square_mean(bin_image)
%필요한 점들 뽑아내기 위한 변수들

rSize = 4;
threshold = 10;    
n = (120/rSize) * (160/rSize); 
ref_image = zeros(120,160);
preporcessingDots = zeros(n,2);
num_dots = 0;

for i=0:((120-rSize)/rSize)
    for j=0:((160-rSize)/rSize)
        if sum(bin_image(rSize*i+1:rSize*i+rSize, rSize*j+1:rSize*j+rSize),'all') > threshold
            ref_image(rSize*i+(rSize/2),rSize*j+(rSize/2))=1;
            num_dots = num_dots+1;
            preporcessingDots(num_dots,1) = rSize*i+(rSize/2);
            preporcessingDots(num_dots,2) = rSize*j+(rSize/2);
        end
    end
end

== matlab function flightControlSystem/Image Processing System/Result of previous work for backup/clustering ==
  data: centroids_before output; X input; centroids output
function [centroids_before,centroids] = fcn(X)



K = 5;
n = size(X, 1);
centroids = zeros(K,2);

% 1st 좌표
centroids(1,:) = [60, 80];

% 2nd  좌표 ,중앙에서 가장 먼 픽셀 찾기
d = 0;
for i = 1:n
   %temp_d = (60-X(i,1))^2  + (80-X(i,2))^2;
   temp_d = norm(centroids(1,:) - X(i,:) );
   if(temp_d > d && X(i,1) ~= 0)
      d= temp_d;
      centroids(2,1) = X(i,1);
      centroids(2,2) = X(i,2);
   end
end

% 3th 좌표
LS=100000;
for i = 1:n
    temp_d1 = norm(centroids(1,:)-X(i,:) );
    temp_d2 = norm(centroids(2,:)-X(i,:) );
    temp_LS = temp_d1^2 + temp_d2^2;
    if((temp_LS < LS) && X(i,1) ~= 0)
        LS = temp_LS;
        centroids(3,1) = X(i,1);
        centroids(3,2) = X(i,2);
   end
end

% 4th, 5th 좌표
LS=100000;
for i = 1:n
    temp_d1 = norm(centroids(1,:)-X(i,:) );
    temp_d3 = norm(centroids(3,:)-X(i,:) );
    temp_LS = temp_d1^2 +  temp_d3^2;
    if((temp_LS < LS) && X(i,1) ~= 0)
        LS = temp_LS;
        centroids(4,1) = X(i,1);
        centroids(4,2) = X(i,2);
    end
end
LS=100000;
for i = 1:n
    temp_d2 = norm(centroids(2,:)-X(i,:) );
    temp_d3 = norm(centroids(3,:)-X(i,:) );
    temp_LS = temp_d2^2 +  temp_d3^2;
    if((temp_LS < LS) && X(i,1) ~= 0)
        LS = temp_LS;
        centroids(5,1) = X(i,1);
        centroids(5,2) = X(i,2);
    end
end
% 6,7,8,9th 좌표는 위에서 한거처럼 하드코딩하면 가능한데 최적화못하겠음.


centroids_before = centroids;


% k-means clustering

% max_iter = 1;
% for i = 1:max_iter
%    % Assign each data point to the closest centroid
%    idx = knnsearch(centroids,X);
%    
%    % Compute new centroids as the mean of the data points in each cluster
%    for k = 1:K
%       centroids(k,:) = mean(X(idx==k,:),1,'omitnan');
%    end
% end
% centroids(isnan(centroids))=0;

idx = knnsearch(centroids,X);
X(X==0) = NaN;
for k = 1:K
      centroids(k,:) = mean(X(idx==k,:),1,'omitnan');
end
centroids(isnan(centroids))=0;

== matlab function flightControlSystem/Image Processing System/Result of previous work for backup/viewer/MATLAB Function1 ==
  data: p input; image output
function image = fcn(p)

image = zeros(120, 160);

for i = 1:5
    if( p(i,1) == 0)  || (p(i,2) == 0)
       continue; 
    end
    x = round(p(i,1));
    y = round(p(i,2));
    image(x,y) = 1;
end

== matlab function flightControlSystem/Image Processing System/Result of previous work for backup/viewer/MATLAB Function2 ==
  data: p input; image output
function image = fcn(p)

image = zeros(120, 160);


for i = 1:5
    if( p(i,1) == 0)  || (p(i,2) == 0)
       continue; 
    end
    x = round(p(i,1));
    y = round(p(i,2));
    image(x,y) = 1;
end

== matlab function flightControlSystem/Image Processing System/landing subsystem/landing check ==
  data: bin_image input; landingFlag output; landingDots output; COG_X parameter; COG_Y parameter; ROI_Size parameter; landingRef output
function [landingFlag, landingDots,landingRef] = fcn(bin_image, COG_X, COG_Y, ROI_Size)

landingFlag = 0;
landingDots = zeros(120*160,2);
landingRef = zeros(1,2);


cnt = 0;
for i = 1:ROI_Size
   for j = 1:ROI_Size
       if bin_image(i,j) == 1
           cnt = cnt + 1;
           landingDots(cnt,1) = i;
           landingDots(cnt,2) = j;
           landingFlag = 1;
       end
   end
end

landingDots(landingDots==0) = NaN;
landingRef = mean(landingDots,1,'omitnan');

landingRef(1) = (ROI_Size/2) - landingRef(1);
landingRef(2) = landingRef(2) - (ROI_Size/2);

== matlab function flightControlSystem/Image Processing System/preprocessing subsystem/image to dots ==
  data: bin_image input; dots output
function dots = fcn(bin_image)

n = 120*160;
dots = zeros(n,2);
num_dots = 0;

for i = 1:120
   for j = 1:160
      if  bin_image(i,j) == 1
          num_dots = num_dots+1;
          dots(num_dots,1) = i;
          dots(num_dots,2) = j;
      end
   end
end

== matlab function flightControlSystem/Image Processing System/Result of previous work for backup/sorting and coordinate_change ==
  data: sortMat output; C input; P output; COG_X parameter; COG_Y parameter
function [ sortMat, P] = fcn(C, COG_X, COG_Y)

K = 5;
sortMat = zeros(K,2);
P = zeros(K,2);
% sorting

d = Inf;
temp_idx = 0;
sortMat(1,:) = C(1,:);
C(1,:) = Inf;
for i = 1:K - 1
    for j = 1:K
       temp_d = norm( sortMat(i,:) - C(j,:) ); 
       if(temp_d < d && temp_d ~= 0)
          d = temp_d;
          sortMat(i+1,:) = C(j,:);
          temp_idx = j;
       end
    end
    if temp_idx ~= 0
        C(temp_idx,:) = Inf;
        d = Inf;
    end
end

% coordinate change
for i = 1:K
   P(i,1) = COG_X - sortMat(i,1);
   P(i,2) = sortMat(i,2) - COG_Y;
end

== matlab function flightControlSystem/Image Processing System/Subsystem/trajectory generation ==
  data: dots input; dx input; dy input; MAP output; centroids_before output; temp_centroids output; COG_X parameter; COG_Y parameter; Points output
function [MAP, centroids_before, temp_centroids, Points]   = fcn(dots, dx, dy, COG_X, COG_Y)


%%%%%%%%%%%%%%%%%  delete tail %%%%%%%%%%%%%%%%% 
num_dots = size(dots,1);
cutting_dots = zeros(num_dots,2);
degree_reange = 45;

% sorting_ref의 두 번째 값을 이전값으로 사용,(일단은 이렇게. 수정이 필요할 수도.)
persistent prev_dx;
persistent prev_dy;

if isempty(prev_dx)
    prev_dx = 0;
end
if isempty(prev_dy)
    prev_dy = 0;
end
%deg = mod( atan2(dy,dx), 2*pi);
%prev_deg = mod(atan2(prev_dy,prev_dx)+pi,2*pi); % 이전 진행 방향 + pi
prev_deg = mod(atan2(dy,dx)+pi,2*pi);

idx = 1;
MAP=zeros(120,160);
for i=1:num_dots
    if abs( mod(atan2(dots(i,2)-COG_Y, COG_X-dots(i,1)),2*pi)  -  prev_deg) > degree_reange*pi/180  &&  dots(i,1) ~= 0
        cutting_dots(idx,1) = dots(i,1);
        cutting_dots(idx,2) = dots(i,2);
        
        MAP(dots(i,1),dots(i,2))=1;
        idx = idx+1;
    end
end

%%%%%%%%%%%%%%% segment processing %%%%%%%%%%%%%%%%




%%%%%%%%%%%%%%%% K-point pick %%%%%%%%%%%%%%%%%%%%%
X = cutting_dots;
K = 5;
n = size(X, 1);
centroids = zeros(K,2);

% 1st 좌표
centroids(1,:) = [60, 80];

% 2nd  좌표 ,중앙에서 가장 먼 픽셀 찾기
d = 0;
for i = 1:n
   %temp_d = (60-X(i,1))^2  + (80-X(i,2))^2;
   temp_d = norm(centroids(1,:) - X(i,:) );
   if(temp_d > d && X(i,1) ~= 0)
      d= temp_d;
      centroids(2,1) = X(i,1);
      centroids(2,2) = X(i,2);
   end
end

% 3th 좌표
LS=100000;
for i = 1:n
    temp_d1 = norm(centroids(1,:)-X(i,:) );
    temp_d2 = norm(centroids(2,:)-X(i,:) );
    temp_LS = temp_d1^2 + temp_d2^2;
    if((temp_LS < LS) && X(i,1) ~= 0)
        LS = temp_LS;
        centroids(3,1) = X(i,1);
        centroids(3,2) = X(i,2);
   end
end

% 4th, 5th 좌표
LS=100000;
for i = 1:n
    temp_d1 = norm(centroids(1,:)-X(i,:) );
    temp_d3 = norm(centroids(3,:)-X(i,:) );
    temp_LS = temp_d1^2 +  temp_d3^2;
    if((temp_LS < LS) && X(i,1) ~= 0)
        LS = temp_LS;
        centroids(4,1) = X(i,1);
        centroids(4,2) = X(i,2);
    end
end
LS=100000;
for i = 1:n
    temp_d2 = norm(centroids(2,:)-X(i,:) );
    temp_d3 = norm(centroids(3,:)-X(i,:) );
    temp_LS = temp_d2^2 +  temp_d3^2;
    if((temp_LS < LS) && X(i,1) ~= 0)
        LS = temp_LS;
        centroids(5,1) = X(i,1);
        centroids(5,2) = X(i,2);
    end
end
% 6,7,8,9th 좌표는 위에서 한거처럼 하드코딩하면 가능한데 최적화못하겠음.

% for viewer
centroids_before = centroids;


%%%%%%%%%%%%%%%%% clustering %%%%%%%%%%%%%%%%% 


idx = knnsearch(centroids,X);
X(X==0) = NaN;
for k = 1:K
      centroids(k,:) = mean(X(idx==k,:),1,'omitnan');
end
centroids(isnan(centroids))=0;

% for viewer
temp_centroids = centroids;

%%%%%%%%%%%%%%%%% sorting %%%%%%%%%%%%%%%%%
sortMat = zeros(K,2);
Points = zeros(K,2);


d = Inf;
temp_idx = 0;
sortMat(1,:) = centroids(1,:);
centroids(1,:) = Inf;
for i = 1:K - 1
    for j = 1:K
       temp_d = norm( sortMat(i,:) - centroids(j,:) ); 
       if(temp_d < d && temp_d ~= 0)
          d = temp_d;
          sortMat(i+1,:) = centroids(j,:);
          temp_idx = j;
       end
    end
    if temp_idx ~= 0
        centroids(temp_idx,:) = Inf;
        d = Inf;
    end
end

%%%%%%%%%%%%%%%%% coordinate change %%%%%%%%%%%%%%%%%
for i = 1:K
   Points(i,1) = COG_X - sortMat(i,1);
   Points(i,2) = sortMat(i,2) - COG_Y;
end

prev_dx = Points(2,1);
prev_dy = Points(2,2);

== matlab function flightControlSystem/Image Processing System/Subsystem/destination point picker ==
  data: u input; y output
function y = fcn(u)

y = u(3,:);
